simulink model "FR"  (R2015b)
settings: Solver=VariableStepAuto  StartTime=0.0  StopTime=10.0  RelTol=1e-3
undefined symbols (not defined in the file): a, alpha, beta, c, Csfr, gama, Ksfr, Kufr, m, Ps, S, tao
settings Model: Creator=Guest  LastModifiedBy=Guest

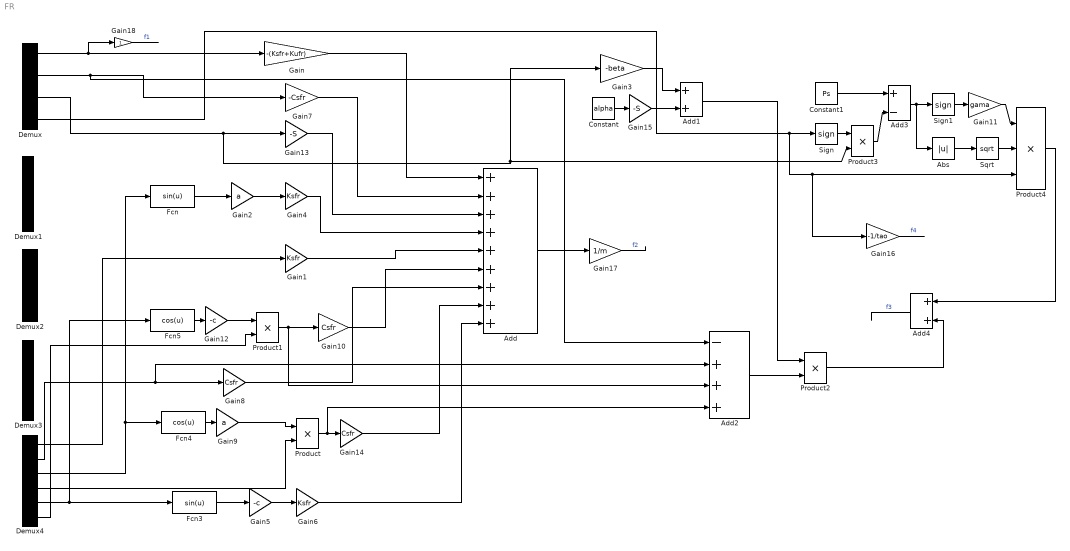
== system FR ==
  Abs : Abs
  Add : Sum  Inputs=+++++++++
  Add1 : Sum
  Add2 : Sum  Inputs=-+++
  Add3 : Sum  Inputs=+-
  Add4 : Sum
  Constant : Constant  Value=alpha
  Constant1 : Constant  Value=Ps
  Demux{,1..3} (4 alike) : Demux
  Demux4 : Demux  Outputs=6
  Fcn : Fcn  Expr=sin(u)
  Fcn3 : Fcn  Expr=sin(u)
  Fcn4 : Fcn  Expr=cos(u)
  Fcn5 : Fcn  Expr=cos(u)
  Gain : Gain  Gain=-(Ksfr+Kufr)
  Gain1 : Gain  Gain=Ksfr
  Gain10 : Gain  Gain=Csfr
  Gain11 : Gain  Gain=gama
  Gain12 : Gain  Gain=-c
  Gain13 : Gain  Gain=-S
  Gain14 : Gain  Gain=Csfr
  Gain15 : Gain  Gain=-S
  Gain16 : Gain  Gain=-1/tao
  Gain17 : Gain  Gain=1/m
  Gain18 : Gain
  Gain2 : Gain  Gain=a
  Gain3 : Gain  Gain=-beta
  Gain4 : Gain  Gain=Ksfr
  Gain5 : Gain  Gain=-c
  Gain6 : Gain  Gain=Ksfr
  Gain7 : Gain  Gain=-Csfr
  Gain8 : Gain  Gain=Csfr
  Gain9 : Gain  Gain=a
  Product{,1..3} (4 alike) : Product
  Product4 : Product  Inputs=3
  Sign : Signum
  Sign1 : Signum
  Sqrt : Sqrt  SaturateOnIntegerOverflow=on
  wires:
  Demux/1 -> Gain18/1, Gain/1
  Demux4/1 -> Gain1/1
  Demux4/3 -> Fcn/1, Fcn4/1
  Fcn/1 -> Gain2/1
  Gain2/1 -> Gain4/1
  Demux4/5 -> Fcn5/1, Fcn3/1
  Fcn3/1 -> Gain5/1
  Gain5/1 -> Gain6/1
  Demux/2 -> Add2/1, Gain7/1
  Demux4/2 -> Add2/2, Gain8/1
  Fcn4/1 -> Gain9/1
  Gain9/1 -> Product/1
  Demux4/4 -> Product/2
  Fcn5/1 -> Gain12/1
  Demux4/6 -> Product1/2
  Gain12/1 -> Product1/1
  Demux/3 -> Gain3/1, Product3/2, Gain13/1
  Gain/1 -> Add/1
  Gain7/1 -> Add/2
  Gain13/1 -> Add/3
  Gain4/1 -> Add/4
  Gain1/1 -> Add/5
  Product1/1 -> Add2/3, Gain10/1
  Gain8/1 -> Add/7
  Product/1 -> Add2/4, Gain14/1
  Gain6/1 -> Add/9
  Constant/1 -> Gain15/1
  Gain3/1 -> Add1/1
  Gain15/1 -> Add1/2
  Gain14/1 -> Add/8
  Gain10/1 -> Add/6
  Add2/1 -> Product2/2
  Add1/1 -> Product2/1
  Demux/4 -> Gain16/1, Product4/3, Sign/1
  Sign/1 -> Product3/1
  Constant1/1 -> Add3/1
  Product3/1 -> Add3/2
  Add3/1 -> Abs/1, Sign1/1
  Sign1/1 -> Gain11/1
  Abs/1 -> Sqrt/1
  Gain11/1 -> Product4/1
  Sqrt/1 -> Product4/2
  Product2/1 -> Add4/2
  Add/1 -> Gain17/1
  Gain17/1 -> ?  "f2"
  Product4/1 -> Add4/1
  Gain18/1 -> ?  "f1"
  Add4/1 -> ?  "f3"
  Gain16/1 -> ?  "f4"
